simulink model "part3_1"  (R2018b)
settings: Solver=VariableStepAuto  StartTime=0.0  StopTime=10.0  RelTol=1e-3
libraries: simulink x1
settings Model: Creator=lisazaher  LastModifiedBy=lisazaher

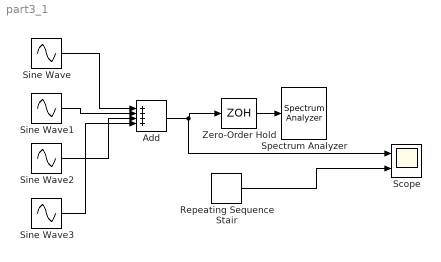
== system part3_1 ==
  Add : Sum  Inputs=++++
  Repeating Sequence Stair : simulink/Sources/Repeating Sequence Stair  OutValues=[-1 1].'  tsamp=1/64  OutMin=[]  OutMax=[]  OutDataTypeStr=double  OutputDataTypeScalingMode=double  OutDataType=fixdt(0,8)  ConRadixGroup=Best Precision: Vector-wise  OutScaling=2^-12
  Scope : Scope  NumInputPorts=2
  Sine Wave : Sin  Amplitude=4/pi  Frequency=64*pi  SampleTime=0
  Sine Wave1 : Sin  Amplitude=4/(3*pi)  Frequency=6*32*pi  SampleTime=0
  Sine Wave2 : Sin  Amplitude=4/(5*pi)  Frequency=10*pi*32  SampleTime=0
  Sine Wave3 : Sin  Amplitude=4/(7*pi)  Frequency=14*pi*32  SampleTime=0
  Spectrum Analyzer : SpectrumAnalyzer
  Zero-Order Hold : ZeroOrderHold  SampleTime=2^-10
  wires:
  Sine Wave/1 -> Add/1
  Sine Wave1/1 -> Add/2
  Sine Wave2/1 -> Add/3
  Sine Wave3/1 -> Add/4
  Add/1 -> Scope/1, Zero-Order Hold/1
  Zero-Order Hold/1 -> Spectrum Analyzer/1
  Repeating Sequence Stair/1 -> Scope/2
